simulink model "Sin_PWM_HBridge_v1"  (Simulink 8.5)
settings: Solver=ode23tb  StartTime=0.0  StopTime=.25  MaxStep=1e-5  RelTol=1e-9
libraries: powerlib x8, powerlib_meascontrol x1
settings Model: Creator=Shailesh  LastModifiedBy=tesla
settings SolverCC: MaxConsecutiveMinStep=20
settings OptimizationCC: InitFltsAndDblsToZero=on
settings DebuggingCC: SaveWithParameterizedLinksMsg=none  SignalResolutionControl=TryResolveAllWithWarning  SolverPrmCheckMsg=warning  MultiTaskDSMMsg=warning  MultiTaskCondExecSysMsg=none  FcnCallInpInsideContextMsg=UseLocalSettings
settings GRTTargetCC: TargetFcnLib=ansi_tfl_tmw.mat

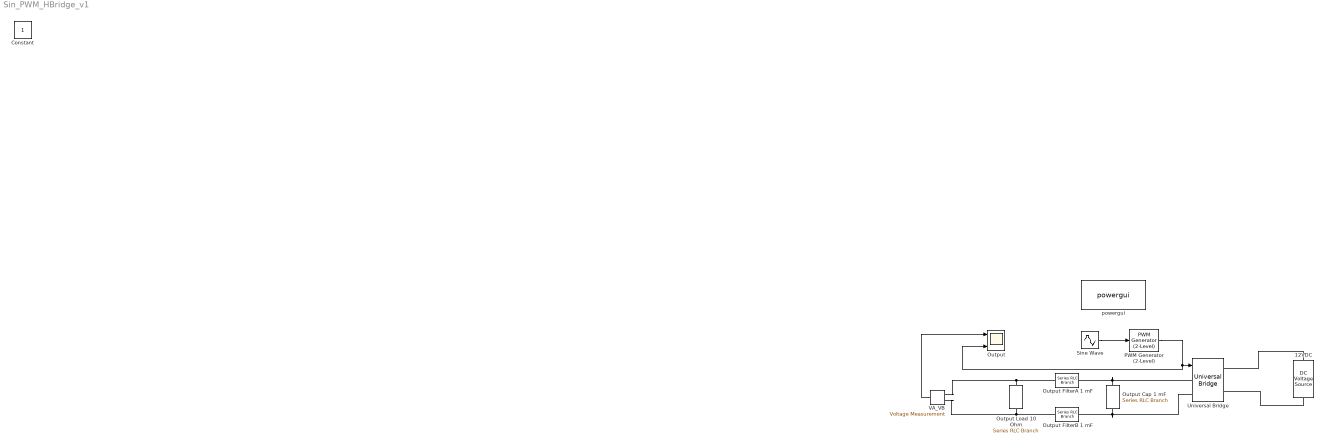
== system Sin_PWM_HBridge_v1 ==
  12VDC : powerlib/Electrical Sources/DC Voltage Source  Amplitude=12  Measurements=None
  Output : Scope  NumInputPorts=2
      settings: YMin=-1~-0.1  YMax=13~1.1  MaxDataPoints=5000000
  Output Cap 1 mF : powerlib/Elements/Series RLC Branch  LConnTagsString=__new0  RConnTagsString=__new0  BranchType=C  Resistance=1  Inductance=1e-3  SetiL0=off  InitialCurrent=0  Capacitance=10e-6  Setx0=off  InitialVoltage=600  Measurements=None
  Output FilterA 1 mF : powerlib/Elements/Series RLC Branch  LConnTagsString=__new0  RConnTagsString=__new0  BranchType=L  Resistance=1  Inductance=1e-3  SetiL0=off  InitialCurrent=0  Capacitance=1e-6  Setx0=off  InitialVoltage=600  Measurements=None
  Output FilterB 1 mF : powerlib/Elements/Series RLC Branch  LConnTagsString=__new0  RConnTagsString=__new0  BranchType=L  Resistance=1  Inductance=1e-3  SetiL0=off  InitialCurrent=0  Capacitance=1e-6  Setx0=off  InitialVoltage=600  Measurements=None
  Output Load 10 Ohm : powerlib/Elements/Series RLC Branch  LConnTagsString=__new0  RConnTagsString=__new0  BranchType=R  Resistance=100  Inductance=1e-3  SetiL0=off  InitialCurrent=0  Capacitance=10e-6  Setx0=off  InitialVoltage=600  Measurements=None
  PWM Generator (2-Level) : powerlib_meascontrol/Pulse & Signal Generators/PWM Generator (2-Level)  ModulatorType=Single-phase full-bridge (4 pulses)  ModulatorMode=Unsynchronized  Fc=30e3  Pc=90  nF=27  MinMax="[ -1  1 ]"  SamplingTechnique=Natural  ModulatingSignals=off  m=0.8  Freq=60  Phase=0  Ts=0  ShowCarrierOutport=off
  Sine Wave : Sin  Amplitude=0.5  Bias=0.5  Frequency=377  SampleTime=0
  Universal Bridge : powerlib/Power Electronics/Universal Bridge  Arms=2  SnubberResistance=1e5  SnubberCapacitance=inf  Device=MOSFET / Diodes  Ron=1e-3  Lon=0  ForwardVoltages="[  0  0  ]"  ForwardVoltage=0  GTOparameters=[ 10e-6 , 20e-6 ]  IGBTparameters=[ 1e-6 , 2e-6 ]  Measurements=None  Measurements_2=None  converterType=Rectifier
  VA_VB : powerlib/Measurements/Voltage Measurement  PhasorSimulation=off  OutputType=Complex  PSBequivalent=0
  powergui : powerlib/powergui  Priority=1  SimulationMode=Continuous  SolverType=Tustin  SampleTime=50e-7  frequency=60  SPID=off  DisableSnubberDevices=off  DisableRonSwitches=off  DisableVfSwitches=off  SwTol=0  DisplayEquations=off  Interpol=off  methode=off  Ts=0  FunctionMessages=off  echomessages=off  HookPort=off  EnableUseOfTLC=off  x0status=blocks  frequencyindice=0  Pbase=100e6  ErrMax=1e-4  Iterations=50  UnitsV=kV  UnitsW=MW  buscounter=0  RestoreLinks=warning  ResistiveCurrentMeasurement=off  Frange=[0:2:500]  Ylog=off  Xlog=on  ShowGrid=off  save=off  variable=ZData  structure=0  ZoomFFT=off  StartTime=0.0  cycles=1  DisplayStyle=1  fundamental=60  FreqAxis=off  MaxFrequency=1000  frequencyindicesteady=1  RmsSteady=1  display=off
  Constant : Constant  IOType=siggen
  wires:
  Sine Wave/1 -> PWM Generator (2-Level)/1
  PWM Generator (2-Level)/1 -> Output/2, Universal Bridge/1
  VA_VB/1 -> Output/1
  connections:
  12VDC/LConn1 -- Universal Bridge/RConn2
  12VDC/RConn1 -- Universal Bridge/RConn1
  Universal Bridge/LConn1 -- Output Cap 1 mF/LConn1 -- Output FilterA 1 mF/LConn1
  Universal Bridge/LConn2 -- Output Cap 1 mF/RConn1 -- Output FilterB 1 mF/LConn1
  Output FilterB 1 mF/RConn1 -- VA_VB/LConn2 -- Output Load 10 Ohm/RConn1
  Output FilterA 1 mF/RConn1 -- VA_VB/LConn1 -- Output Load 10 Ohm/LConn1
